simulink model "seno"  (R2022a)
settings: Solver=ode4  StartTime=0.0  StopTime=10.0  FixedStep=0.01  RelTol=1e-3
settings Model: Creator=leonardonavacastellanos  LastModifiedBy=leonardonavacastellanos

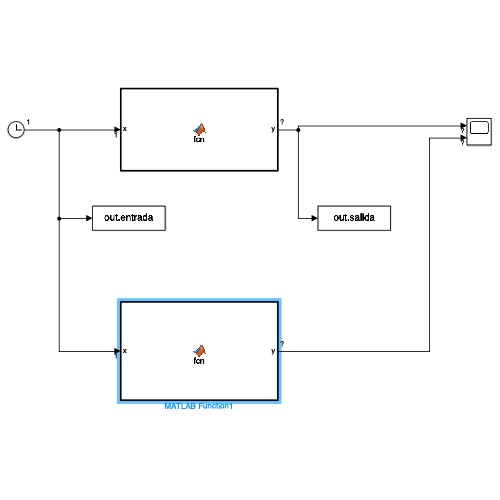
[thumbnail: Simulink's stored preview of the top-level diagram]
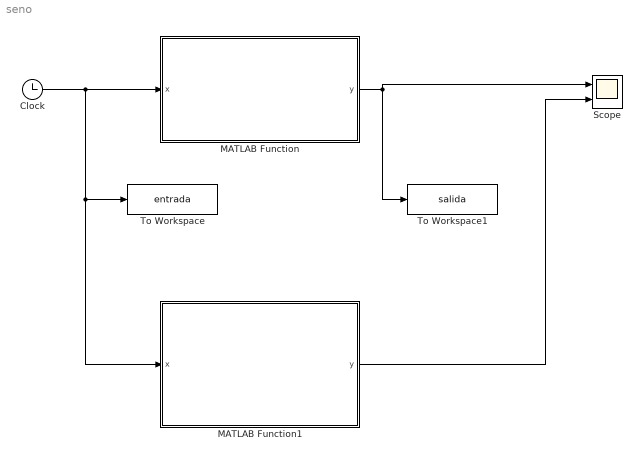
== system seno ==
  Clock : Clock
  MATLAB Function : MATLAB Function  TreatAsAtomicUnit=on
  MATLAB Function1 : MATLAB Function  TreatAsAtomicUnit=on
  Scope : Scope  NumInputPorts=2
  To Workspace : ToWorkspace  VariableName=entrada  SampleTime=-1
      settings: Save2DSignal=2-D array (concatenate along first dimension)
  To Workspace1 : ToWorkspace  VariableName=salida  SampleTime=-1
      settings: Save2DSignal=2-D array (concatenate along first dimension)
  wires:
  Clock/1 -> MATLAB Function/1(x), MATLAB Function1/1(x), To Workspace/1
  MATLAB Function/1(y) -> Scope/1, To Workspace1/1
  MATLAB Function1/1(y) -> Scope/2

== matlab function seno/MATLAB Function ==
  data: x input; y output
function y = fcn(x)

y = sin(x);

== matlab function seno/MATLAB Function1 ==
  data: x input; y output
function y = fcn(x)

X = [-17.502756752362065648310235575879;
    -17.502756752362065648310235575879;
    -17.502756752362065648310235575879;
    -17.502756752362065648310235575879;
    -17.502756752362065648310235575879;
    -17.502756752362065648310235575879;
    -17.502756752362065648310235575879;
    -17.502756752362065648310235575879;
    -17.502756752362065648310235575879;
    6.7203175936673055247913874307332;
    6.7203175936673055247913874307332;
    6.7203175936673055247913874307332;
    6.7203175936673055247913874307332;
    6.7203175936673055247913874307332;
    6.7203175936673055247913874307332;
    6.7203175936673055247913874307332;
    6.7203175936673055247913874307332;
    6.7203175936673055247913874307332;
    -9.5967892946264378033598642429751;
    -9.5967892946264378033598642429751;
    -9.5967892946264378033598642429751;
    -9.5967892946264378033598642429751;
    -9.5967892946264378033598642429751;
    -9.5967892946264378033598642429751;
    -9.5967892946264378033598642429751;
    -9.5967892946264378033598642429751;
    -9.5967892946264378033598642429751;
    0.15945254379305529006879775705681];

w1 = X(1);
w2 = X(2);
w3 = X(3);
w4 = X(4);
w5 = X(5);
w6 = X(6);
w7 = X(7);
w8 = X(8);
w9 = X(9);
w10 = X(10);
w11 = X(11);
w12 = X(12);
w13 = X(13);
w14 = X(14);
w15 = X(15);
w16 = X(16);
w17 = X(17);
w18 = X(18);
b1 = X(19);
b2 = X(20);
b3 = X(21);
b4 = X(22);
b5 = X(23);
b6 = X(24);
b7 = X(25);
b8 = X(26);
b9 = X(27);
b10 = X(28);

disp(w1)

y = (w10/(1 + exp(-(w1*x + b1)))) + (w11/(1 + exp(-(w2*x + b2)))) + (w12/(1 + exp(-(w3*x + b3)))) + (w13/(1 + exp(-(w4*x + b4)))) + (w14/(1 + exp(-(w5*x + b5)))) + (w15/(1 + exp(-(w6*x + b6)))) + (w16/(1 + exp(-(w7*x + b7)))) + (w17/(1 + exp(-(w8*x + b8)))) + (w18/(1 + exp(-(w9*x + b9)))) + b10 ;
